simulink model "zynqRadioHWSWQPSKAD9361AD9364SL"  (R2025a)
settings: Solver=FixedStepDiscrete  StartTime=0.0  StopTime=0.5  RelTol=1e-3
PreLoadFcn:
  | setTxBurstLength = 10000;
  | txtmsg = ['Zynq radio HW/SW Co-design ÞÞÞÞ']; % Use only printable characters
  | 
  | %------------------------------------------------------------------------------------------------------
  | if ~isequal(size(txtmsg),[1 31])
  |     error('txtmsg must contain 31 characters');
  | end
  | 
  | [dataBits,msg] = zynqRadioHWSWQPSKgenHelloworldMsg(20); % generate 20 msgs for LUT
  | msgLUT = uint8(msg);
  | dataBitsLUT = dataBits(:);
  | Rsym                = 10e3;%1.92e6;
  | Config = zynqRadioHWSWQPSKTxRxParameters;
  | fs = Rsym*Config.SamplesPerSymbol;
  | word = [txtmsg newline];  % append a new line character to txtmsg
  | 
  | % The highest clock rate is 16 times the message character rate.
  | % As the message characters are fed at highest clock to FPGA
  | % repeat each character 16 times to maintain the message rate.
  | word = repelem(word.',16,1);
  | repeatTimes = ceil(setTxBurstLength/length(word));
  | inpData = complex(repmat(uint8(word),repeatTimes,1));
  | inUseTxBurstLength = length(inpData);
PostLoadFcn:
  | hScopeConfig = get_param([gcs '/HDL_QPSK/QPSK Tx Channel QPSK Rx/QPSK Rx/Frequency and Time Synchronizer/Symbol Synchronizer/No HDL/QPSK Receiver Eye Diagram'],'ScopeConfiguration');
  | hScopeConfig.OpenAtSimulationStart = false;
  | hScopeConfig.Visible = false;
  | clear hScopeConfig
InitFcn:
  | setTxBurstLength = 10000;
  | txtmsg = ['Zynq radio HW/SW Co-design ÞÞÞÞ']; % Use only printable characters
  | 
  | %------------------------------------------------------------------------------------------------------
  | if ~isequal(size(txtmsg),[1 31])
  |     error('txtmsg must contain 31 characters');
  | end
  | 
  | [dataBits,msg] = zynqRadioHWSWQPSKgenHelloworldMsg(20); % generate 20 msgs for LUT
  | msgLUT = uint8(msg);
  | dataBitsLUT = dataBits(:);
  | Rsym                = 10e3;%1.92e6;
  | Config = zynqRadioHWSWQPSKTxRxParameters;
  | fs = Rsym*Config.SamplesPerSymbol;
  | word = [txtmsg newline];  % append a new line character to txtmsg
  | 
  | % The highest clock rate is 16 times the message character rate.
  | % As the message characters are fed at highest clock to FPGA
  | % repeat each character 16 times to maintain the message rate.
  | word = repelem(word.',16,1);
  | repeatTimes = ceil(setTxBurstLength/length(word));
  | inpData = complex(repmat(uint8(word),repeatTimes,1));
  | inUseTxBurstLength = length(inpData);
  | 
  | Config.Preamble = logical(zeros(0,1))
undefined symbols (not defined in the file or in its folder): Add, dspblkCoreblockFVToolHelper, gcbh, gse_genframes, Shift
libraries: hdlsllib x144, simulink x37, dsphdlsigops2 x3, dsphdlfiltering2 x3, whdlutilities x3, dsphdlxfrm2 x2, dsphdlmathfun2 x2, commdigbbndpm3 x2, sdrzblksprivate x1
(part 4 of 6)

== system zynqRadioHWSWQPSKAD9361AD9364SL/HDL_QPSK/QPSK Tx Channel QPSK Rx/QPSK Rx/Frequency and Time Synchronizer/Preamble Detector/Timing Adjust ==
  timingOffset : Inport
  timingOffsetValid : Inport  Port=2
  dataIn : Inport  Port=3
  validIn : Inport  Port=4
  Delay{,1..4} (5 alike) : Delay  DelayLength=1
  Logical Operator : Logic  AllPortsSameDT=off  OutDataTypeStr=boolean
  Logical Operator1 : Logic  Operator=NOT  AllPortsSameDT=off  OutDataTypeStr=boolean
  Logical Operator2 : Logic  Inputs=3  AllPortsSameDT=off  OutDataTypeStr=boolean
  No HDL : Subsystem
  Relational Operator : RelationalOperator  Operator===  OutDataTypeStr=boolean  InputSameDT=off
  State Register : hdlsllib/Discrete/Unit Delay Enabled Resettable Synchronous  InitialCondition=0.0  SampleTime=-1
  Unit Delay Enabled Synchronous3 : hdlsllib/Discrete/Unit Delay Enabled Synchronous  InitialCondition=0.0  SampleTime=-1
  timing Reference : hdlsllib/Sources/HDL Counter  CountType=Count limited  CountInit=0  CountStep=1  CountMax=searchSamples - 1  CountFromType=Initial value  CountFrom=0  CountResetPort=off  CountLoadPort=off  CountEnbPort=on  CountDirPort=off  CountHitOutputPort=off  CountDataType=Unsigned  CountWordLen=nextpow2(searchSamples - 1)  CountFracLen=0  CountSampTime=1
  dataOut : Outport
  validOut : Outport  Port=2
  SyncPulse : Outport  Port=3
  wires:
  Delay4/1 -> dataOut/1
  Delay3/1 -> validOut/1
  timingOffset/1 -> Unit Delay Enabled Synchronous3/1
  Unit Delay Enabled Synchronous3/1 -> Relational Operator/2
  Delay/1 -> SyncPulse/1
  validIn/1 -> timing Reference/1, Logical Operator2/1, No HDL/1(validIn), Delay3/1
  State Register/1 -> Logical Operator2/3, Delay1/1
  Logical Operator1/1 -> Logical Operator/2
  Relational Operator/1 -> Logical Operator2/2
  Logical Operator2/1 -> No HDL/3(syncPulse), Delay/1, Delay2/1
  Delay2/1 -> State Register/3
  Logical Operator/1 -> State Register/1, State Register/2, Unit Delay Enabled Synchronous3/2
  timing Reference/1 -> No HDL/2(timingOffset), Relational Operator/1
  timingOffsetValid/1 -> Logical Operator/1
  Delay1/1 -> Logical Operator1/1
  dataIn/1 -> Delay4/1

== system zynqRadioHWSWQPSKAD9361AD9364SL/HDL_QPSK/QPSK Tx Channel QPSK Rx/QPSK Rx/Frequency and Time Synchronizer/Symbol Synchronizer/Gardner TED ==
  data : Inport
  strobe : Inport  Port=2
  Constant : Constant  Value=0  OutDataTypeStr=Inherit: Inherit via back propagation  SampleTime=1/(Rsym*SamplesPerSymbol)
  Delay10 : Delay  DelayLength=4
  GTED : Subsystem
  Switch : Switch  Criteria=u2 ~= 0  InputSameDT=off
  e : Outport  VectorParamsAs1DForOutWhenUnconnected=off
  wires:
  Constant/1 -> Switch/3
  Switch/1 -> e/1
  strobe/1 -> Delay10/1
  data/1 -> GTED/1(In1)
  GTED/1(Out1) -> Switch/1
  Delay10/1 -> Switch/2

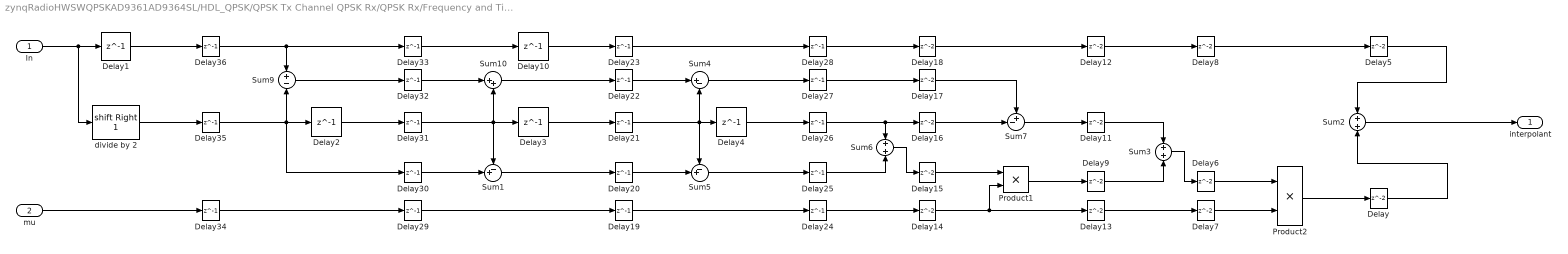
== system zynqRadioHWSWQPSKAD9361AD9364SL/HDL_QPSK/QPSK Tx Channel QPSK Rx/QPSK Rx/Frequency and Time Synchronizer/Symbol Synchronizer/Interpolation Filter ==
  In : Inport
  mu : Inport  Port=2
  Delay{,5..9,11..18} (14 alike) : Delay
  Delay{1..4,10} (5 alike) : Delay  DelayLength=1  InitialCondition=0
  Delay{19..36} (18 alike) : Delay  DelayLength=1
  Product1 : Product  OutDataTypeStr=fixdt(1,16,10)  RndMeth=Zero
  Product2 : Product  RndMeth=Zero  OutDataTypeStr=Inherit: Same as first input
  Sum1 : Sum  Inputs=-+|
  Sum10 : Sum  Inputs=|++
  Sum2 : Sum  Inputs=+|+
  Sum3 : Sum  Inputs=+|+  OutDataTypeStr=fixdt(1,16,10)
  Sum4 : Sum  Inputs=|+-
  Sum5 : Sum  Inputs=-+|
  Sum6 : Sum  Inputs=+|+  OutDataTypeStr=fixdt(1,16,11)  SaturateOnIntegerOverflow=on
  Sum7 : Sum  Inputs=+-|  OutDataTypeStr=fixdt(1,16,10)
  Sum9 : Sum  Inputs=+-
  divide by 2 : ArithShift  BitShiftNumber=1  BitShiftDirection=Right
  interpolant : Outport
  wires:
  Sum9/1 -> Delay32/1
  In/1 -> divide by 2/1, Delay1/1
  Sum2/1 -> interpolant/1
  Sum7/1 -> Delay11/1
  Product1/1 -> Delay9/1
  Product2/1 -> Delay/1
  Sum3/1 -> Delay6/1
  Sum1/1 -> Delay20/1
  Delay3/1 -> Delay21/1
  Sum10/1 -> Delay22/1
  Delay2/1 -> Delay31/1
  Delay1/1 -> Delay36/1
  divide by 2/1 -> Delay35/1
  Delay/1 -> Sum2/2
  Delay5/1 -> Sum2/1
  Delay6/1 -> Product2/1
  Delay7/1 -> Product2/2
  Delay8/1 -> Delay5/1
  Delay9/1 -> Sum3/2
  Delay11/1 -> Sum3/1
  Delay12/1 -> Delay8/1
  Delay13/1 -> Delay7/1
  Delay14/1 -> Delay13/1, Product1/2
  Delay15/1 -> Product1/1
  Delay16/1 -> Sum7/2
  Delay17/1 -> Sum7/1
  Delay18/1 -> Delay12/1
  mu/1 -> Delay34/1
  Sum5/1 -> Delay25/1
  Delay4/1 -> Delay26/1
  Sum4/1 -> Delay27/1
  Delay10/1 -> Delay23/1
  Delay24/1 -> Delay14/1
  Sum6/1 -> Delay15/1
  Delay26/1 -> Delay16/1, Sum6/1
  Delay27/1 -> Delay17/1
  Delay28/1 -> Delay18/1
  Delay25/1 -> Sum6/2
  Delay19/1 -> Delay24/1
  Delay20/1 -> Sum5/2
  Delay21/1 -> Sum4/2, Sum5/1, Delay4/1
  Delay22/1 -> Sum4/1
  Delay23/1 -> Delay28/1
  Delay29/1 -> Delay19/1
  Delay30/1 -> Sum1/2
  Delay31/1 -> Sum1/1, Sum10/2, Delay3/1
  Delay32/1 -> Sum10/1
  Delay33/1 -> Delay10/1
  Delay34/1 -> Delay29/1
  Delay35/1 -> Delay30/1, Delay2/1, Sum9/2
  Delay36/1 -> Delay33/1, Sum9/1

== system zynqRadioHWSWQPSKAD9361AD9364SL/HDL_QPSK/QPSK Tx Channel QPSK Rx/QPSK Rx/Frequency and Time Synchronizer/Symbol Synchronizer/Loop Filter ==
  note: Proportional-Plus-Integrator Loop Filter,
      | Infinite DC Response to guarantee convergence
  e : Inport
  Add : Sum
  Add2 : Sum  Inputs=|++  OutDataTypeStr=Inherit: Same as first input
  Data Type Conversion17 : DataTypeConversion  OutDataTypeStr=fixdt(1,11,10)  SaturateOnIntegerOverflow=off  RndMeth=Floor
  Delay : Delay  DelayLength=1
  Delay1 : Delay  DelayLength=1  InitialCondition=0
  Delay2 : Delay  InitialCondition=0
  Delay3 : Delay  InitialCondition=0
  Delay4 : Delay  DelayLength=1  InitialCondition=0
  Delay5 : Delay  InitialCondition=0
  Delay6 : Delay  DelayLength=1
  K1 : Gain  Gain=fi(SSLoopFilterPropGain,1,24,24)  ParamDataTypeStr=Inherit: Inherit from 'Gain'  OutDataTypeStr=fixdt(1,30,23)
  K2 : Gain  Gain=fi(SSLoopFilterIntegGain,1,24,24)  ParamDataTypeStr=Inherit: Inherit from 'Gain'  OutDataTypeStr=fixdt(1,30,23)
  v : Outport
  wires:
  Delay/1 -> Add2/2
  Delay5/1 -> Delay6/1
  Delay3/1 -> Delay1/1
  e/1 -> Delay2/1
  Add/1 -> Data Type Conversion17/1
  Delay1/1 -> Add/1
  Delay4/1 -> Add/2
  Delay2/1 -> K1/1, K2/1
  Data Type Conversion17/1 -> v/1
  K2/1 -> Delay5/1
  Add2/1 -> Delay/1, Delay4/1
  K1/1 -> Delay3/1
  Delay6/1 -> Add2/1

== system zynqRadioHWSWQPSKAD9361AD9364SL/HDL_QPSK/QPSK Tx Channel QPSK Rx/QPSK Rx/Frequency and Time Synchronizer/Symbol Synchronizer/No HDL ==
  data : Inport
  valid : Inport  Port=2
  Data Type Conversion : DataTypeConversion  OutDataTypeStr=double  SaturateOnIntegerOverflow=off  RndMeth=Floor
  No HDL : Subsystem
  QPSK Receiver Eye Diagram : EyeDiagramBlock  WindowPosition=[177.000000,528.000000,1920.000000,977.000000,]  ScopeFrameLocation=window  SamplesPerSymbol=SamplesPerSymbol  SymbolsPerTrace=1  Title=RRC Matched Filtered Output  YLimits=[-1.1602,1.2629]
      settings: OpenAtSimulationStart=off
  Unit Delay Enabled Synchronous : hdlsllib/Discrete/Unit Delay Enabled Synchronous  InitialCondition=0.0  SampleTime=-1
  wires:
  data/1 -> No HDL/1(data), Unit Delay Enabled Synchronous/1
  Data Type Conversion/1 -> QPSK Receiver Eye Diagram/1
  Unit Delay Enabled Synchronous/1 -> Data Type Conversion/1
  valid/1 -> Unit Delay Enabled Synchronous/2, No HDL/Enable

== system zynqRadioHWSWQPSKAD9361AD9364SL/HDL_QPSK/QPSK Tx Channel QPSK Rx/QPSK Rx/Frequency and Time Synchronizer/Symbol Synchronizer/Rate Handle ==
  dataIn : Inport
  strobe : Inport  Port=2
  validIn : Inport  Port=3
  Compare To Constant : simulink/Logic and Bit Operations/Compare To Constant  relop===  const=0  OutDataTypeStr=boolean
  Constant : Constant  Value=false  SampleTime=-1
  FIFO : Subsystem  mask{fifoSize=32*4, pushFullDiag=Error, popEmptyDiag=Ignore}
      mask prompts: fifoSize "FIFO size:"; pushFullDiag "Push full FIFO:"; popEmptyDiag "Pop empty FIFO:"
      mask TypeOptions pushFullDiag: Ignore | Warning | Error
      mask TypeOptions popEmptyDiag: Ignore | Warning | Error
  HDL Counter : hdlsllib/Sources/HDL Counter  CountType=Count limited  CountInit=0  CountStep=1  CountMax=SamplesPerSymbol - 1  CountFromType=Initial value  CountFrom=0  CountResetPort=off  CountLoadPort=off  CountEnbPort=on  CountDirPort=off  CountHitOutputPort=off  CountDataType=Unsigned  CountWordLen=nextpow2(SamplesPerSymbol - 1)  CountFracLen=0  CountSampTime=1
  Logical Operator : Logic  AllPortsSameDT=off  OutDataTypeStr=boolean
  Logical Operator1 : Logic  AllPortsSameDT=off  OutDataTypeStr=boolean
  Terminator : Terminator
  dataOut : Outport
  validOut : Outport  Port=2
  wires:
  dataIn/1 -> FIFO/1(in)
  validIn/1 -> Logical Operator1/2, Logical Operator/1, HDL Counter/1
  HDL Counter/1 -> Compare To Constant/1
  Compare To Constant/1 -> Logical Operator/2
  Logical Operator/1 -> FIFO/3(pop)
  FIFO/1(out) -> dataOut/1
  FIFO/3(validPop) -> validOut/1
  FIFO/2(numEntries) -> Terminator/1  "rx_fts_ss_rh_fifo_numEntries"
  Constant/1 -> FIFO/4(reset)
  strobe/1 -> Logical Operator1/1
  Logical Operator1/1 -> FIFO/2(push)

== system zynqRadioHWSWQPSKAD9361AD9364SL/HDL_QPSK/QPSK Tx Channel QPSK Rx/QPSK Tx/Bit Packetizer/Data Bits FIFO/No HDL ==
  push : Inport
  pop : Inport  Port=2
  MATLAB Function : MATLAB Function  TreatAsAtomicUnit=on
  No HDL : Subsystem
  wires:
  push/1 -> MATLAB Function/1(wr), No HDL/1(push)
  pop/1 -> MATLAB Function/2(rd), No HDL/5(pop)
  MATLAB Function/2(ncount) -> No HDL/3(ncount)
  MATLAB Function/1(full) -> No HDL/2(full)
  MATLAB Function/3(empty) -> No HDL/4(empty)

== system zynqRadioHWSWQPSKAD9361AD9364SL/HDL_QPSK/QPSK Tx Channel QPSK Rx/QPSK Tx/Bit Packetizer/Preamble Bits Generator/Preamble Bits Store ==
  note: The Preamble is padded with zeros in the LUT such that
      | the length is the 2^nextpow2(length(Preamble)) for
      | efficient resource mapping to RAM
  actualPreamble : Inport
  sampleCount : Inport  Port=2
  Constant : Constant  OutDataTypeStr=boolean  SampleTime=1/(Rsym*4)
  Extract Bits : simulink/Logic and Bit Operations/Extract Bits  bitsToExtract=Range of bits  numBits=8  bitIdxRange=[0 nextpow2(length(Preamble))-1]  outScalingMode=Treat bit field as an integer
  Preamble : LookupNDDirect  NumberOfTableDimensions=1  Table=[Preamble;false(32-length(Preamble),1)]  DiagnosticForOutOfRangeInput=Error
  Switch : Switch  Criteria=u2 ~= 0  Threshold=1  SaturateOnIntegerOverflow=off  InputSameDT=off
  preamble : Outport
  wires:
  Switch/1 -> preamble/1
  Constant/1 -> Switch/3
  Extract Bits/1 -> Preamble/1
  Preamble/1 -> Switch/1
  sampleCount/1 -> Extract Bits/1
  actualPreamble/1 -> Switch/2

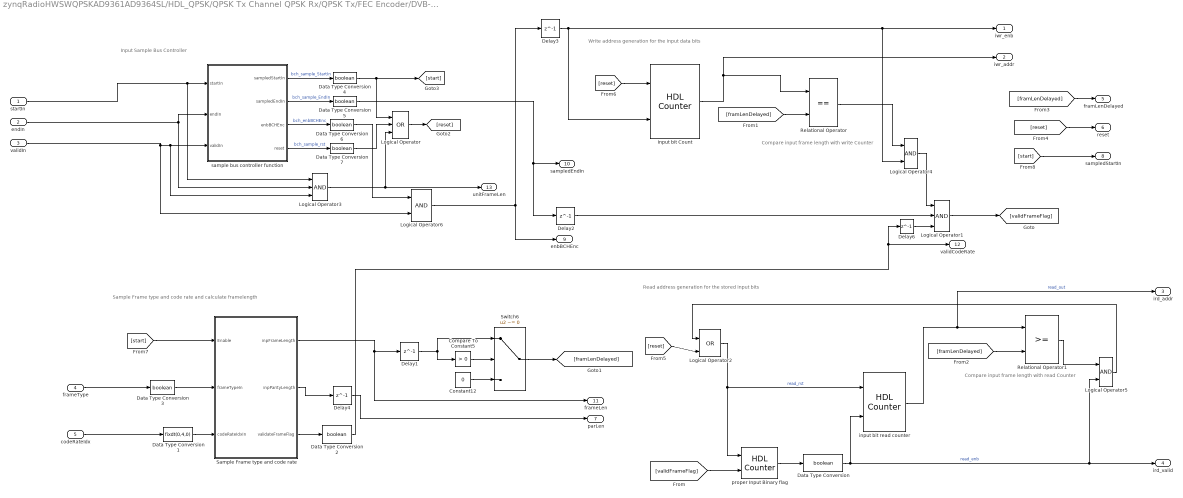
== system zynqRadioHWSWQPSKAD9361AD9364SL/HDL_QPSK/QPSK Tx Channel QPSK Rx/QPSK Tx/FEC Encoder/DVB-S2 BCH Encoder/Input controller ==
  note: Input Sample Bus Controller
  note: Compare input frame length with read Counter
  note: Compare input frame length with write Counter
  note: Sample Frame type and code rate and calculate framelength
  note: Write address generation for the input data bits
  note: Read address generation for the stored input bits
  startIn : Inport
  endIn : Inport  Port=2
  validIn : Inport  Port=3
  frameType : Inport  Port=4
  codeRateIdx : Inport  Port=5
  Compare To Constant5 : simulink/Logic and Bit Operations/Compare To Constant  relop=>  const=0  OutDataTypeStr=boolean
  Constant12 : Constant  Value=0  OutDataTypeStr=Inherit: Inherit via back propagation  SampleTime=-1
  Data Type Conversion{,2,4..7} (6 alike) : DataTypeConversion  OutDataTypeStr=boolean  SaturateOnIntegerOverflow=off  RndMeth=Floor
  Data Type Conversion1 : DataTypeConversion  OutDataTypeStr=fixdt(0,4,0)  RndMeth=Nearest  SaturateOnIntegerOverflow=off
  Data Type Conversion3 : DataTypeConversion  OutDataTypeStr=boolean  RndMeth=Nearest  SaturateOnIntegerOverflow=off
  Delay{1..4,6} (5 alike) : Delay  DelayLength=1
  Input bit Count : hdlsllib/Sources/HDL Counter  CountType=Count limited  CountInit=0  CountStep=1  CountMax=65535  CountFromType=Initial value  CountFrom=0  CountResetPort=on  CountLoadPort=off  CountEnbPort=on  CountDirPort=off  CountHitOutputPort=off  CountDataType=Unsigned  CountWordLen=16  CountFracLen=0  CountSampTime=1
  Logical Operator : Logic  Operator=OR  Inputs=3  IconShape=distinctive  AllPortsSameDT=off  OutDataTypeStr=boolean
  Logical Operator1 : Logic  Inputs=3  IconShape=distinctive  AllPortsSameDT=off  OutDataTypeStr=boolean
  Logical Operator2 : Logic  Operator=OR  IconShape=distinctive  AllPortsSameDT=off  OutDataTypeStr=boolean
  Logical Operator3 : Logic  Inputs=3  IconShape=distinctive  AllPortsSameDT=off  OutDataTypeStr=boolean
  Logical Operator4 : Logic  IconShape=distinctive  AllPortsSameDT=off  OutDataTypeStr=boolean
  Logical Operator5 : Logic  IconShape=distinctive  AllPortsSameDT=off  OutDataTypeStr=boolean
  Logical Operator6 : Logic  IconShape=distinctive  AllPortsSameDT=off  OutDataTypeStr=boolean
  Relational Operator : RelationalOperator  Operator===  OutDataTypeStr=boolean  InputSameDT=off
  Relational Operator1 : RelationalOperator  OutDataTypeStr=boolean  InputSameDT=off
  Sample Frame type and code rate : MATLAB Function  TreatAsAtomicUnit=on
  Switch6 : Switch  Criteria=u2 ~= 0  SaturateOnIntegerOverflow=off  InputSameDT=off
  input bit read counter : hdlsllib/Sources/HDL Counter  CountType=Count limited  CountInit=0  CountStep=1  CountMax=65535  CountFromType=Initial value  CountFrom=0  CountResetPort=on  CountLoadPort=off  CountEnbPort=on  CountDirPort=off  CountHitOutputPort=off  CountDataType=Unsigned  CountWordLen=16  CountFracLen=0  CountSampTime=1
  proper Input Binary flag : hdlsllib/Sources/HDL Counter  CountType=Count limited  CountInit=0  CountStep=1  CountMax=1  CountFromType=Initial value  CountFrom=0  CountResetPort=on  CountLoadPort=off  CountEnbPort=on  CountDirPort=off  CountHitOutputPort=off  CountDataType=Unsigned  CountWordLen=1  CountFracLen=0  CountSampTime=1
  sample bus controller function : MATLAB Function  TreatAsAtomicUnit=on
  iwr_enb : Outport
  iwr_addr : Outport  Port=2
  ird_addr : Outport  Port=3
  ird_valid : Outport  Port=4
  framLenDelayed : Outport  Port=5
  reset : Outport  Port=6
  parLen : Outport  Port=7
  sampledStartIn : Outport  Port=8
  enbBCHEnc : Outport  Port=9
  sampledEndIn : Outport  Port=10
  frameLen : Outport  Port=11
  validCodeRate : Outport  Port=12
  unitFrameLen : Outport  Port=13
  wires:
  Input bit Count/1 -> iwr_addr/1, Relational Operator/1
  Data Type Conversion2/1 -> Delay6/1, validCodeRate/1
  input bit read counter/1 -> ird_addr/1, Relational Operator1/1  "read_out"
  Data Type Conversion/1 -> input bit read counter/2, Logical Operator5/2, ird_valid/1  "read_enb"
  Sample Frame type and code rate/1(inpFrameLength) -> frameLen/1, Delay1/1
  Delay3/1 -> iwr_enb/1, Logical Operator4/2, Input bit Count/2
  Logical Operator3/1 -> Logical Operator/3, unitFrameLen/1
  Delay4/1 -> parLen/1
  [validFrameFlag] -> proper Input Binary flag/2
  Delay6/1 -> Logical Operator1/3
  Sample Frame type and code rate/3(validateFrameFlag) -> Data Type Conversion2/1
  Relational Operator1/1 -> Logical Operator5/1
  Relational Operator/1 -> Logical Operator4/1
  Sample Frame type and code rate/2(inpParityLength) -> Delay4/1
  Logical Operator5/1 -> Logical Operator2/1
  Logical Operator2/1 -> proper Input Binary flag/1, input bit read counter/1  "read_rst"
  proper Input Binary flag/1 -> Data Type Conversion/1
  Logical Operator1/1 -> [validFrameFlag]
  Delay2/1 -> Logical Operator1/2
  Data Type Conversion5/1 -> Delay2/1, sampledEndIn/1
  Delay1/1 -> Compare To Constant5/1, Switch6/1
  Data Type Conversion4/1 -> [start], Logical Operator/1
  Logical Operator6/1 -> enbBCHEnc/1, Delay3/1
  codeRateIdx/1 -> Data Type Conversion1/1
  frameType/1 -> Data Type Conversion3/1
  Data Type Conversion1/1 -> Sample Frame type and code rate/3(codeRateIdxIn)
  Logical Operator4/1 -> Logical Operator1/1
  Data Type Conversion3/1 -> Sample Frame type and code rate/2(frameTypeIn)
  Constant12/1 -> Switch6/3
  Compare To Constant5/1 -> Switch6/2
  Data Type Conversion6/1 -> Logical Operator6/1
  Data Type Conversion7/1 -> Logical Operator/2
  startIn/1 -> Logical Operator3/1, sample bus controller function/1(startIn)
  validIn/1 -> Logical Operator6/2, Logical Operator3/3, sample bus controller function/3(validIn)
  sample bus controller function/2(sampledEndIn) -> Data Type Conversion5/1  "bch_sample_EndIn"
  sample bus controller function/3(enbBCHEnc) -> Data Type Conversion6/1  "bch_enbBCHEnc"
  endIn/1 -> sample bus controller function/2(endIn), Logical Operator3/2
  sample bus controller function/4(reset) -> Data Type Conversion7/1  "bch_sample_rst"
  sample bus controller function/1(sampledStartIn) -> Data Type Conversion4/1  "bch_sample_StartIn"
  Switch6/1 -> [framLenDelayed]
  [framLenDelayed] -> Relational Operator/2
  [framLenDelayed] -> Relational Operator1/2
  [framLenDelayed] -> framLenDelayed/1
  Logical Operator/1 -> [reset]
  [reset] -> reset/1
  [reset] -> Logical Operator2/2
  [reset] -> Input bit Count/1
  [start] -> Sample Frame type and code rate/1(Enable)
  [start] -> sampledStartIn/1

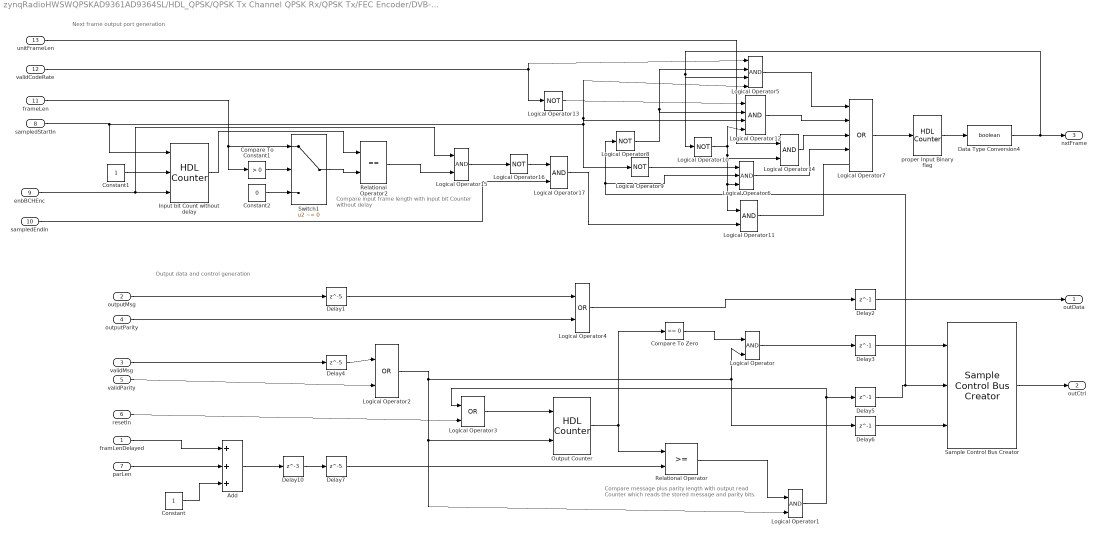
== system zynqRadioHWSWQPSKAD9361AD9364SL/HDL_QPSK/QPSK Tx Channel QPSK Rx/QPSK Tx/FEC Encoder/DVB-S2 BCH Encoder/Output Controller ==
  note: Output data and control generation
  note: Next frame output port generation
  note: Compare message plus parity length with output read Counter which reads the stored message and parity bits.
  note: Compare input frame length with input bit Counter without delay
  framLenDelayed : Inport
  outputMsg : Inport  Port=2
  validMsg : Inport  Port=3
  outputParity : Inport  Port=4
  validParity : Inport  Port=5
  resetIn : Inport  Port=6
  parLen : Inport  Port=7
  sampledStartIn : Inport  Port=8
  enbBCHEnc : Inport  Port=9
  sampledEndIn : Inport  Port=10
  frameLen : Inport  Port=11
  validCodeRate : Inport  Port=12
  unitFrameLen : Inport  Port=13
  Add : Sum  Inputs=+++  OutDataTypeStr=Inherit: Same as first input
  Compare To Constant1 : simulink/Logic and Bit Operations/Compare To Constant  relop=>  const=0  OutDataTypeStr=boolean
  Compare To Zero : hdlsllib/Logic and Bit Operations/Compare To Zero  relop===  OutDataTypeStr=boolean
  Constant : Constant  OutDataTypeStr=Inherit: Inherit via back propagation  SampleTime=-1
  Constant1 : Constant  OutDataTypeStr=uint16  SampleTime=-1
  Constant2 : Constant  Value=0  OutDataTypeStr=Inherit: Inherit via back propagation  SampleTime=-1
  Data Type Conversion4 : DataTypeConversion  OutDataTypeStr=boolean  SaturateOnIntegerOverflow=off  RndMeth=Floor
  Delay1 : Delay  DelayLength=5
  Delay10 : Delay  DelayLength=3
  Delay{2..3,5..6} (4 alike) : Delay  DelayLength=1
  Delay4 : Delay  DelayLength=5
  Delay7 : Delay  DelayLength=5
  "Input bit Count without delay " : hdlsllib/Sources/HDL Counter  CountType=Count limited  CountInit=0  CountStep=1  CountMax=65535  CountFromType=Initial value  CountFrom=0  CountResetPort=off  CountLoadPort=on  CountEnbPort=on  CountDirPort=off  CountHitOutputPort=off  CountDataType=Unsigned  CountWordLen=16  CountFracLen=0  CountSampTime=1
  Logical Operator{,1,11,14..15,17} (6 alike) : Logic  IconShape=distinctive  AllPortsSameDT=off  OutDataTypeStr=boolean
  Logical Operator{8..10,13,16} (5 alike) : Logic  Operator=NOT  IconShape=distinctive  AllPortsSameDT=off  OutDataTypeStr=boolean
  Logical Operator12 : Logic  Inputs=4  IconShape=distinctive  AllPortsSameDT=off  OutDataTypeStr=boolean
  Logical Operator2 : Logic  Operator=OR  IconShape=distinctive  AllPortsSameDT=off  OutDataTypeStr=boolean
  Logical Operator3 : Logic  Operator=OR  IconShape=distinctive  AllPortsSameDT=off  OutDataTypeStr=boolean
  Logical Operator4 : Logic  Operator=OR  IconShape=distinctive  AllPortsSameDT=off  OutDataTypeStr=boolean
  Logical Operator5 : Logic  Inputs=4  IconShape=distinctive  AllPortsSameDT=off  OutDataTypeStr=boolean
  Logical Operator6 : Logic  Inputs=3  IconShape=distinctive  AllPortsSameDT=off  OutDataTypeStr=boolean
  Logical Operator7 : Logic  Operator=OR  Inputs=5  IconShape=distinctive  AllPortsSameDT=off  OutDataTypeStr=boolean
  Output Counter : hdlsllib/Sources/HDL Counter  CountType=Count limited  CountInit=0  CountStep=1  CountMax=65535  CountFromType=Initial value  CountFrom=0  CountResetPort=on  CountLoadPort=off  CountEnbPort=on  CountDirPort=off  CountHitOutputPort=off  CountDataType=Unsigned  CountWordLen=16  CountFracLen=0  CountSampTime=1
  Relational Operator : RelationalOperator  OutDataTypeStr=boolean  InputSameDT=off
  Relational Operator2 : RelationalOperator  Operator===  OutDataTypeStr=boolean  InputSameDT=off
  Sample Control Bus Creator : whdlutilities/Sample Control Bus Creator
  Switch1 : Switch  Criteria=u2 ~= 0  SaturateOnIntegerOverflow=off  InputSameDT=off
  proper Input Binary flag : hdlsllib/Sources/HDL Counter  CountType=Count limited  CountInit=1  CountStep=1  CountMax=0  CountFromType=Initial value  CountFrom=1  CountResetPort=off  CountLoadPort=off  CountEnbPort=on  CountDirPort=off  CountHitOutputPort=off  CountDataType=Unsigned  CountWordLen=1  CountFracLen=0  CountSampTime=1
  outData : Outport
  outCtrl : Outport  Port=2
  nxtFrame : Outport  Port=3
  wires:
  Logical Operator/1 -> Delay3/1
  Logical Operator4/1 -> Delay2/1
  Sample Control Bus Creator/1 -> outCtrl/1
  resetIn/1 -> Logical Operator3/2
  Output Counter/1 -> Relational Operator/1, Compare To Zero/1
  Compare To Zero/1 -> Logical Operator/1
  Logical Operator3/1 -> Output Counter/1
  Logical Operator1/1 -> Logical Operator3/1, Delay5/1
  Relational Operator/1 -> Logical Operator1/1
  validParity/1 -> Logical Operator2/2
  Logical Operator2/1 -> Logical Operator1/2, Output Counter/2, Delay6/1, Logical Operator/2
  outputParity/1 -> Logical Operator4/2
  Delay1/1 -> Logical Operator4/1
  Delay4/1 -> Logical Operator2/1
  Delay2/1 -> outData/1
  Delay3/1 -> Sample Control Bus Creator/1
  Delay5/1 -> Logical Operator6/2, Logical Operator8/1, Sample Control Bus Creator/2
  Delay6/1 -> Sample Control Bus Creator/3
  Delay7/1 -> Relational Operator/2
  proper Input Binary flag/1 -> Data Type Conversion4/1
  Data Type Conversion4/1 -> nxtFrame/1, Logical Operator10/1, Logical Operator5/3
  Logical Operator7/1 -> proper Input Binary flag/1
  Logical Operator8/1 -> Logical Operator12/2, Logical Operator5/2
  Logical Operator9/1 -> Logical Operator6/1
  Logical Operator10/1 -> Logical Operator12/4, Logical Operator14/2, Logical Operator11/1, Logical Operator6/3
  Logical Operator6/1 -> Logical Operator7/4
  Logical Operator5/1 -> Logical Operator7/1
  outputMsg/1 -> Delay1/1
  validMsg/1 -> Delay4/1
  Delay10/1 -> Delay7/1
  Logical Operator17/1 -> Logical Operator11/2
  Logical Operator11/1 -> Logical Operator7/5
  validCodeRate/1 -> Logical Operator5/1, Logical Operator13/1
  Logical Operator12/1 -> Logical Operator7/2
  Logical Operator13/1 -> Logical Operator12/1
  parLen/1 -> Add/2
  unitFrameLen/1 -> Logical Operator14/1
  Logical Operator14/1 -> Logical Operator7/3
  Constant/1 -> Add/3
  framLenDelayed/1 -> Add/1
  Add/1 -> Delay10/1
  sampledStartIn/1 -> "Input bit Count without delay "/1, Logical Operator5/4, Logical Operator12/3, Logical Operator9/1
  enbBCHEnc/1 -> Logical Operator15/1, "Input bit Count without delay "/3
  frameLen/1 -> Compare To Constant1/1, Switch1/1
  Constant1/1 -> "Input bit Count without delay "/2
  Relational Operator2/1 -> Logical Operator15/2
  Compare To Constant1/1 -> Switch1/2
  Constant2/1 -> Switch1/3
  Logical Operator16/1 -> Logical Operator17/1
  sampledEndIn/1 -> Logical Operator17/2
  "Input bit Count without delay "/1 -> Relational Operator2/1
  Switch1/1 -> Relational Operator2/2
  Logical Operator15/1 -> Logical Operator16/1

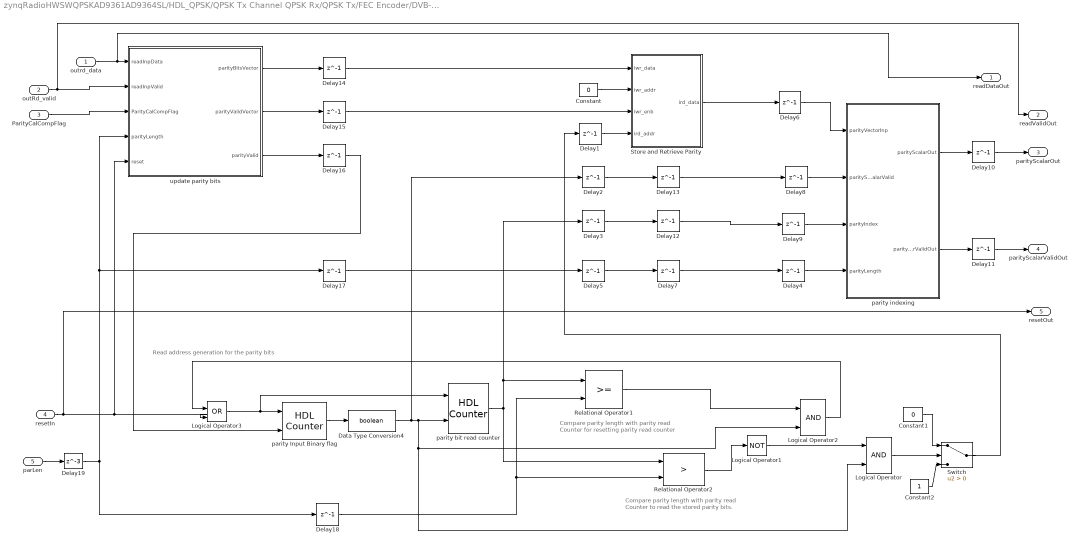
== system zynqRadioHWSWQPSKAD9361AD9364SL/HDL_QPSK/QPSK Tx Channel QPSK Rx/QPSK Tx/FEC Encoder/DVB-S2 BCH Encoder/Parity Generation ==
  note: Read address generation for the parity bits
  note: Compare parity length with parity read Counter for resetting parity read counter
  note: Compare parity length with parity read Counter to read the stored parity bits.
  outrd_data : Inport
  outRd_valid : Inport  Port=2
  ParityCalCompFlag : Inport  Port=3
  resetIn : Inport  Port=4
  parLen : Inport  Port=5
  Constant : Constant  Value=0  VectorParams1D=off  OutDataTypeStr=fixdt(0,3,0)  SampleTime=-1
  Constant1 : Constant  Value=0  VectorParams1D=off  OutDataTypeStr=fixdt(0,3,0)  SampleTime=-1
  Constant2 : Constant  VectorParams1D=off  OutDataTypeStr=fixdt(0,3,0)  SampleTime=-1
  Data Type Conversion4 : DataTypeConversion  OutDataTypeStr=boolean  SaturateOnIntegerOverflow=off  RndMeth=Floor
  Delay{1..18} (18 alike) : Delay  DelayLength=1
  Delay19 : Delay  DelayLength=3
  Logical Operator : Logic  IconShape=distinctive  AllPortsSameDT=off  OutDataTypeStr=boolean
  Logical Operator1 : Logic  Operator=NOT  IconShape=distinctive  AllPortsSameDT=off  OutDataTypeStr=boolean
  Logical Operator2 : Logic  IconShape=distinctive  AllPortsSameDT=off  OutDataTypeStr=boolean
  Logical Operator3 : Logic  Operator=OR  IconShape=distinctive  AllPortsSameDT=off  OutDataTypeStr=boolean
  Relational Operator1 : RelationalOperator  OutDataTypeStr=boolean  InputSameDT=off
  Relational Operator2 : RelationalOperator  Operator=>  OutDataTypeStr=boolean  InputSameDT=off
  Store and Retrieve Parity : Subsystem  TreatAsAtomicUnit=on
      settings: LibrarySourceBlock=|
      | hdlsllib/Ports &
      | Subsystems/For Each
      | Subsystem
  Switch : Switch  Criteria=u2 > Threshold  SaturateOnIntegerOverflow=off  InputSameDT=off
  parity Input Binary flag : hdlsllib/Sources/HDL Counter  CountType=Count limited  CountInit=0  CountStep=1  CountMax=1  CountFromType=Initial value  CountFrom=0  CountResetPort=on  CountLoadPort=off  CountEnbPort=on  CountDirPort=off  CountHitOutputPort=off  CountDataType=Unsigned  CountWordLen=1  CountFracLen=0  CountSampTime=1
  parity bit read counter : hdlsllib/Sources/HDL Counter  CountType=Count limited  CountInit=0  CountStep=1  CountMax=255  CountFromType=Initial value  CountFrom=0  CountResetPort=on  CountLoadPort=off  CountEnbPort=on  CountDirPort=off  CountHitOutputPort=off  CountDataType=Unsigned  CountWordLen=8  CountFracLen=0  CountSampTime=1
  parity indexing : MATLAB Function  TreatAsAtomicUnit=on
  update parity bits : MATLAB Function  TreatAsAtomicUnit=on
  readDataOut : Outport
  readValidOut : Outport  Port=2
  parityScalarOut : Outport  Port=3
  parityScalarValidOut : Outport  Port=4
  resetOut : Outport  Port=5
  wires:
  Logical Operator1/1 -> Logical Operator/1
  parity Input Binary flag/1 -> Data Type Conversion4/1
  Relational Operator1/1 -> Logical Operator2/1
  Logical Operator3/1 -> parity Input Binary flag/1, parity bit read counter/1
  Constant2/1 -> Switch/3
  Constant1/1 -> Switch/1
  Logical Operator2/1 -> Logical Operator3/1
  Relational Operator2/1 -> Logical Operator1/1
  Logical Operator/1 -> Switch/2
  Delay10/1 -> parityScalarOut/1
  Delay11/1 -> parityScalarValidOut/1
  update parity bits/3(parityValid) -> Delay16/1
  update parity bits/1(parityBitsVector) -> Delay14/1
  outRd_valid/1 -> readValidOut/1, update parity bits/2(readInpValid)
  outrd_data/1 -> readDataOut/1, update parity bits/1(readInpData)
  Store and Retrieve Parity/1(ird_data) -> Delay6/1
  Constant/1 -> Store and Retrieve Parity/2(iwr_addr)
  update parity bits/2(parityValidVector) -> Delay15/1
  ParityCalCompFlag/1 -> update parity bits/3(ParityCalCompFlag)
  Switch/1 -> Delay1/1
  parity indexing/2(parityScalarValidOut) -> Delay11/1
  parity indexing/1(parityScalarOut) -> Delay10/1
  parLen/1 -> Delay19/1
  parity bit read counter/1 -> Relational Operator1/1, Delay3/1, Relational Operator2/1
  Data Type Conversion4/1 -> Logical Operator/2, Logical Operator2/2, parity bit read counter/2, Delay2/1
  resetIn/1 -> resetOut/1, update parity bits/5(reset), Logical Operator3/2
  Delay1/1 -> Store and Retrieve Parity/4(ird_addr)
  Delay2/1 -> Delay13/1
  Delay3/1 -> Delay12/1
  Delay4/1 -> parity indexing/4(parityLength)
  Delay5/1 -> Delay7/1
  Delay6/1 -> parity indexing/1(parityVectorInp)
  Delay7/1 -> Delay4/1
  Delay8/1 -> parity indexing/2(parityScalarValid)
  Delay9/1 -> parity indexing/3(parityIndex)
  Delay13/1 -> Delay8/1
  Delay12/1 -> Delay9/1
  Delay14/1 -> Store and Retrieve Parity/1(iwr_data)
  Delay15/1 -> Store and Retrieve Parity/3(iwr_enb)
  Delay16/1 -> parity Input Binary flag/2
  Delay17/1 -> Delay5/1
  Delay18/1 -> Relational Operator1/2, Relational Operator2/2
  Delay19/1 -> Delay18/1, Delay17/1, update parity bits/4(parityLength)

== system zynqRadioHWSWQPSKAD9361AD9364SL/HDL_QPSK/QPSK Tx Channel QPSK Rx/QPSK Tx/FEC Encoder/DVB-S2 BCH Encoder/Store and Retreive Input ==
  note: write and read input data using RAM
  note: Compare input frame length with read Counter
  iwr_data : Inport
  iwr_enb : Inport  Port=2
  iwr_addr : Inport  Port=3
  ird_addr : Inport  Port=4
  ird_valid : Inport  Port=5
  framLenDelayed : Inport  Port=6
  resetIn : Inport  Port=7
  Constant : Constant  Value=0  OutDataTypeStr=Inherit: Inherit via back propagation  SampleTime=-1
  Constant2 : Constant  Value=0  OutDataTypeStr=Inherit: Inherit via back propagation  SampleTime=-1
  Data RAM : hdlsllib/HDL RAMs/Simple Dual Port RAM  ram_size=16
  Data Type Duplicate : DataTypeDuplicate
  Data Type Duplicate1 : DataTypeDuplicate
  Data Type Conversion : DataTypeConversion  OutDataTypeStr=boolean  SaturateOnIntegerOverflow=off  RndMeth=Floor
  Delay{,1..3,7} (5 alike) : Delay  DelayLength=1
  Delay4 : Delay
  Delay5 : Delay
  Delay6 : Delay
  Logical Operator : Logic  Operator=NOT  IconShape=distinctive  AllPortsSameDT=off  OutDataTypeStr=boolean
  Logical Operator1 : Logic  IconShape=distinctive  AllPortsSameDT=off  OutDataTypeStr=boolean
  Logical Operator2 : Logic  IconShape=distinctive  AllPortsSameDT=off  OutDataTypeStr=boolean
  Relational Operator1 : RelationalOperator  OutDataTypeStr=boolean  InputSameDT=off
  Switch : Switch  Criteria=u2 > Threshold  SaturateOnIntegerOverflow=off  InputSameDT=off
  Switch1 : Switch  Criteria=u2 ~= 0  SaturateOnIntegerOverflow=off  InputSameDT=off
  framLenDelay : Outport
  outrd_data : Outport  Port=2
  outRd_valid : Outport  Port=3
  ParityCalCompFlag : Outport  Port=4
  resetOut : Outport  Port=5
  wires:
  Data RAM/1 -> Delay4/1
  iwr_data/1 -> Delay7/1
  ird_valid/1 -> Delay/1
  framLenDelayed/1 -> framLenDelay/1, Delay2/1
  Delay1/1 -> Relational Operator1/1
  Delay2/1 -> Relational Operator1/2
  Relational Operator1/1 -> Logical Operator1/1
  Logical Operator1/1 -> Delay6/1
  resetIn/1 -> resetOut/1, Logical Operator/1
  Logical Operator/1 -> Delay3/1
  Logical Operator2/1 -> Delay5/1, Logical Operator1/2
  Delay/1 -> Logical Operator2/1
  Delay3/1 -> Logical Operator2/2
  Switch/1 -> outrd_data/1
  Delay5/1 -> Switch/2, outRd_valid/1
  Delay6/1 -> ParityCalCompFlag/1
  Delay4/1 -> Switch/1, Data Type Duplicate/1
  Constant/1 -> Switch/3, Data Type Duplicate/2
  Switch1/1 -> Data RAM/1
  ird_addr/1 -> Data RAM/4, Delay1/1
  iwr_enb/1 -> Data RAM/3, Switch1/2
  iwr_addr/1 -> Data RAM/2
  Data Type Conversion/1 -> Switch1/1, Data Type Duplicate1/1
  Constant2/1 -> Data Type Duplicate1/2, Switch1/3
  Delay7/1 -> Data Type Conversion/1

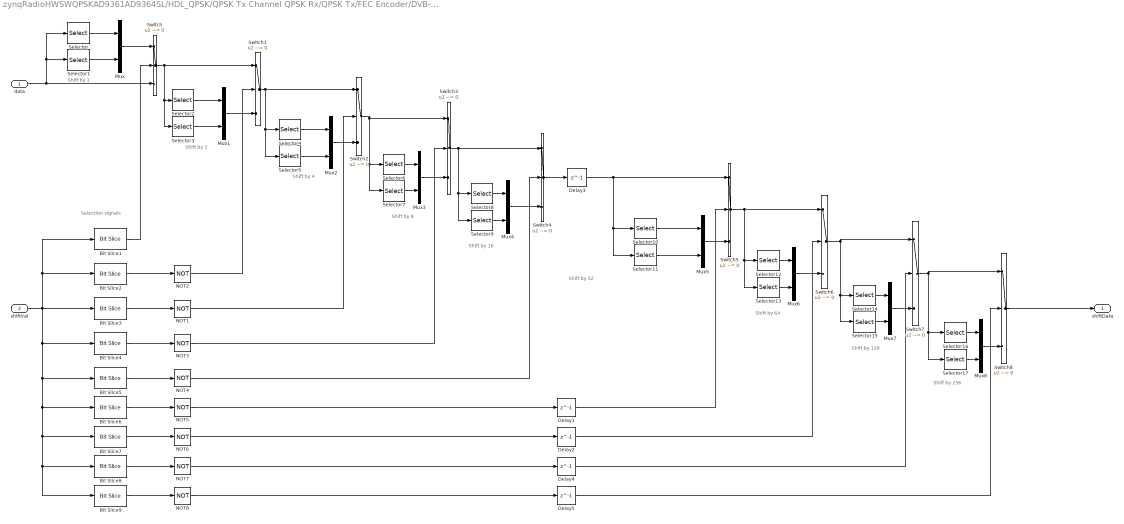
== system zynqRadioHWSWQPSKAD9361AD9364SL/HDL_QPSK/QPSK Tx Channel QPSK Rx/QPSK Tx/FEC Encoder/DVB-S2 LDPC Encoder/Circular Shifter ==
  note: Shift by 256
  note: Shift by 128
  note: Shift by 64
  note: Shift by 32
  note: Shift by 16
  note: Shift by 8
  note: Shift by 4
  note: Shift by 2
  note: Shift by 1
  note: Selection signals
  data : Inport
  shiftVal : Inport  Port=2
  Bit Slice1 : hdlsllib/Logic and Bit Operations/Bit Slice  lidx=0  ridx=0
  Bit Slice2 : hdlsllib/Logic and Bit Operations/Bit Slice  lidx=1  ridx=1
  Bit Slice3 : hdlsllib/Logic and Bit Operations/Bit Slice  lidx=2  ridx=2
  Bit Slice4 : hdlsllib/Logic and Bit Operations/Bit Slice  lidx=3  ridx=3
  Bit Slice5 : hdlsllib/Logic and Bit Operations/Bit Slice  lidx=4  ridx=4
  Bit Slice6 : hdlsllib/Logic and Bit Operations/Bit Slice  lidx=5  ridx=5
  Bit Slice7 : hdlsllib/Logic and Bit Operations/Bit Slice  lidx=6  ridx=6
  Bit Slice8 : hdlsllib/Logic and Bit Operations/Bit Slice  lidx=7  ridx=7
  Bit Slice9 : hdlsllib/Logic and Bit Operations/Bit Slice  lidx=8  ridx=8
  Delay{1..5} (5 alike) : Delay  DelayLength=1
  Mux{,1..8} (9 alike) : Mux  Inputs=2
  NOT{1..8} (8 alike) : Logic  Operator=NOT  IconShape=distinctive  AllPortsSameDT=off  OutDataTypeStr=boolean
  Selector : Selector  InputPortWidth=360  IndexOptions=Index vector (dialog)  Indices=[2 : 360]  OutputSizes=1
  Selector1 : Selector  InputPortWidth=360  IndexOptions=Index vector (dialog)  Indices=[1]  OutputSizes=1
  Selector10 : Selector  InputPortWidth=360  IndexOptions=Index vector (dialog)  Indices=[33: 360]  OutputSizes=1
  Selector11 : Selector  InputPortWidth=360  IndexOptions=Index vector (dialog)  Indices=[1:32]  OutputSizes=1
  Selector12 : Selector  InputPortWidth=360  IndexOptions=Index vector (dialog)  Indices=[65: 360]  OutputSizes=1
  Selector13 : Selector  InputPortWidth=360  IndexOptions=Index vector (dialog)  Indices=[1:64]  OutputSizes=1
  Selector14 : Selector  InputPortWidth=360  IndexOptions=Index vector (dialog)  Indices=[129: 360]  OutputSizes=1
  Selector15 : Selector  InputPortWidth=360  IndexOptions=Index vector (dialog)  Indices=[1:128]  OutputSizes=1
  Selector16 : Selector  InputPortWidth=360  IndexOptions=Index vector (dialog)  Indices=[257: 360]  OutputSizes=1
  Selector17 : Selector  InputPortWidth=360  IndexOptions=Index vector (dialog)  Indices=[1:256]  OutputSizes=1
  Selector2 : Selector  InputPortWidth=360  IndexOptions=Index vector (dialog)  Indices=[3 : 360]  OutputSizes=1
  Selector3 : Selector  InputPortWidth=360  IndexOptions=Index vector (dialog)  Indices=[1:2]  OutputSizes=1
  Selector4 : Selector  InputPortWidth=360  IndexOptions=Index vector (dialog)  Indices=[5 : 360]  OutputSizes=1
  Selector5 : Selector  InputPortWidth=360  IndexOptions=Index vector (dialog)  Indices=[1:4]  OutputSizes=1
  Selector6 : Selector  InputPortWidth=360  IndexOptions=Index vector (dialog)  Indices=[9 : 360]  OutputSizes=1
  Selector7 : Selector  InputPortWidth=360  IndexOptions=Index vector (dialog)  Indices=[1:8]  OutputSizes=1
  Selector8 : Selector  InputPortWidth=360  IndexOptions=Index vector (dialog)  Indices=[17 : 360]  OutputSizes=1
  Selector9 : Selector  InputPortWidth=360  IndexOptions=Index vector (dialog)  Indices=[1:16]  OutputSizes=1
  Switch{,1..8} (9 alike) : Switch  Criteria=u2 ~= 0  InputSameDT=off
  shiftData : Outport
  wires:
  Delay5/1 -> Switch8/2
  Delay4/1 -> Switch7/2
  Delay2/1 -> Switch6/2
  Delay1/1 -> Switch5/2
  Delay3/1 -> Switch5/1, Selector10/1, Selector11/1
  NOT8/1 -> Delay5/1
  NOT7/1 -> Delay4/1
  NOT6/1 -> Delay2/1
  NOT5/1 -> Delay1/1
  Switch4/1 -> Delay3/1
  NOT4/1 -> Switch4/2
  NOT3/1 -> Switch3/2
  NOT1/1 -> Switch2/2
  NOT2/1 -> Switch1/2
  Bit Slice1/1 -> Switch/2
  Bit Slice9/1 -> NOT8/1
  Bit Slice8/1 -> NOT7/1
  Bit Slice7/1 -> NOT6/1
  Bit Slice6/1 -> NOT5/1
  Bit Slice5/1 -> NOT4/1
  Bit Slice4/1 -> NOT3/1
  Bit Slice3/1 -> NOT1/1
  Bit Slice2/1 -> NOT2/1
  Mux8/1 -> Switch8/3
  Switch7/1 -> Switch8/1, Selector17/1, Selector16/1
  Selector16/1 -> Mux8/1
  Selector17/1 -> Mux8/2
  Mux7/1 -> Switch7/3
  Selector15/1 -> Mux7/2
  Switch6/1 -> Switch7/1, Selector15/1, Selector14/1
  Selector14/1 -> Mux7/1
  Mux6/1 -> Switch6/3
  Switch5/1 -> Switch6/1, Selector13/1, Selector12/1
  Selector13/1 -> Mux6/2
  Selector12/1 -> Mux6/1
  Selector10/1 -> Mux5/1
  Mux5/1 -> Switch5/3
  Selector11/1 -> Mux5/2
  Mux4/1 -> Switch4/3
  Selector8/1 -> Mux4/1
  Switch3/1 -> Selector9/1, Selector8/1, Switch4/1
  Selector9/1 -> Mux4/2
  Mux3/1 -> Switch3/3
  Switch2/1 -> Switch3/1, Selector7/1, Selector6/1
  Selector7/1 -> Mux3/2
  Selector6/1 -> Mux3/1
  Switch1/1 -> Selector5/1, Selector4/1, Switch2/1
  Selector4/1 -> Mux2/1
  Mux2/1 -> Switch2/3
  Selector5/1 -> Mux2/2
  Mux1/1 -> Switch1/3
  Switch/1 -> Switch1/1, Selector2/1, Selector3/1
  Selector2/1 -> Mux1/1
  Selector3/1 -> Mux1/2
  Selector1/1 -> Mux/2
  Selector/1 -> Mux/1
  Mux/1 -> Switch/1
  data/1 -> Switch/3, Selector1/1, Selector/1
  shiftVal/1 -> Bit Slice9/1, Bit Slice8/1, Bit Slice7/1, Bit Slice6/1, Bit Slice5/1, Bit Slice4/1, Bit Slice3/1, Bit Slice2/1, Bit Slice1/1
  Switch8/1 -> shiftData/1

== system zynqRadioHWSWQPSKAD9361AD9364SL/HDL_QPSK/QPSK Tx Channel QPSK Rx/QPSK Tx/FEC Encoder/DVB-S2 LDPC Encoder/Input RAM ==
  iwr_data : Inport
  iwr_addr : Inport  Port=2
  iwr_enb : Inport  Port=3
  ird_addr : Inport  Port=4
  AND : Logic  IconShape=distinctive  AllPortsSameDT=off  OutDataTypeStr=boolean
  ConvertToMux : MATLAB Function  TreatAsAtomicUnit=on
  ConvertToWord : MATLAB Function  TreatAsAtomicUnit=on
  Data Type Conversion{,1..3} (4 alike) : DataTypeConversion  OutDataTypeStr=fixdt(0,1,0)  SaturateOnIntegerOverflow=off  RndMeth=Floor
  Delay : Delay  DelayLength=1
  Delay1 : Delay  DelayLength=1
  Dual Port RAM System{,1..3} (4 alike) : hdlsllib/HDL RAMs/Dual Port RAM System  RAMType=Simple dual port  AsyncRead=off  WriteOutputValue=New data  RAMInitialValue=0  allowBusInputs=off  WritesHaveOutput=on  NumReads=0  NumWrites=1  SimulateUsing=Code generation  ModelRAMDelay=on  VectorAccess=Parallel
  Mux : Mux
  Relational Operator : RelationalOperator  Operator===  OutDataTypeStr=boolean  RndMeth=Simplest  InputSameDT=off
  Selector : Selector  InputPortWidth=360  IndexOptions=Index vector (dialog)  Indices=[1:90]  OutputSizes=1
  Selector1 : Selector  InputPortWidth=360  IndexOptions=Index vector (dialog)  Indices=[91:180]  OutputSizes=1
  Selector2 : Selector  InputPortWidth=360  IndexOptions=Index vector (dialog)  Indices=[181:270]  OutputSizes=1
  Selector3 : Selector  InputPortWidth=360  IndexOptions=Index vector (dialog)  Indices=[271:360]  OutputSizes=1
  Switch : Switch  Criteria=u2 > Threshold  SaturateOnIntegerOverflow=off  InputSameDT=off
  ird_data : Outport
  wires:
  Mux/1 -> Switch/3
  ConvertToMux/3(y3) -> Mux/3
  Dual Port RAM System1/1 -> ConvertToMux/2(u2)
  ConvertToMux/1(y1) -> Mux/1
  ConvertToWord/2(y2) -> Dual Port RAM System1/1
  ConvertToWord/4(y4) -> Dual Port RAM System2/1
  ird_addr/1 -> Dual Port RAM System/4, Relational Operator/2, Dual Port RAM System1/4, Dual Port RAM System3/4, Dual Port RAM System2/4
  Data Type Conversion2/1 -> ConvertToWord/3(u3)
  Dual Port RAM System3/1 -> ConvertToMux/3(u3)
  Delay1/1 -> AND/2
  Data Type Conversion/1 -> ConvertToWord/1(u1)
  Selector/1 -> Data Type Conversion/1
  Switch/1 -> ird_data/1
  Data Type Conversion1/1 -> ConvertToWord/2(u2)
  Delay/1 -> Switch/1
  ConvertToWord/1(y1) -> Dual Port RAM System/1
  AND/1 -> Switch/2
  ConvertToMux/4(y4) -> Mux/4
  iwr_addr/1 -> Dual Port RAM System/2, Dual Port RAM System1/2, Dual Port RAM System2/2, Dual Port RAM System3/2, Relational Operator/1
  Data Type Conversion3/1 -> ConvertToWord/4(u4)
  Dual Port RAM System2/1 -> ConvertToMux/4(u4)
  iwr_enb/1 -> Dual Port RAM System/3, Dual Port RAM System1/3, Dual Port RAM System3/3, Dual Port RAM System2/3, Delay1/1
  Selector2/1 -> Data Type Conversion2/1
  ConvertToWord/3(y3) -> Dual Port RAM System3/1
  Dual Port RAM System/1 -> ConvertToMux/1(u1)
  ConvertToMux/2(y2) -> Mux/2
  Relational Operator/1 -> AND/1
  iwr_data/1 -> Selector/1, Selector1/1, Selector2/1, Selector3/1, Delay/1
  Selector3/1 -> Data Type Conversion3/1
  Selector1/1 -> Data Type Conversion1/1

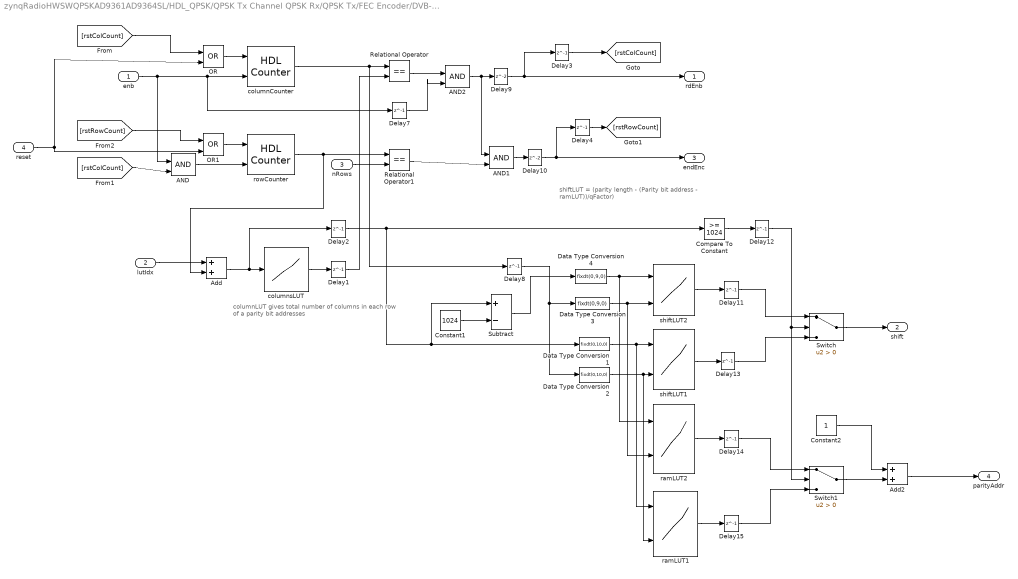
== system zynqRadioHWSWQPSKAD9361AD9364SL/HDL_QPSK/QPSK Tx Channel QPSK Rx/QPSK Tx/FEC Encoder/DVB-S2 LDPC Encoder/Parity Address Generator ==
  note: shiftLUT = (parity length - (Parity bit address -
      | ramLUT))/qFactor)
  note: columnLUT gives total number of columns
      | in each row of a parity bit addresses
  enb : Inport
  lutIdx : Inport  Port=2
  nRows : Inport  Port=3
  reset : Inport  Port=4
  AND : Logic  IconShape=distinctive  AllPortsSameDT=off  OutDataTypeStr=boolean
  AND1 : Logic  IconShape=distinctive  AllPortsSameDT=off  OutDataTypeStr=boolean
  AND2 : Logic  IconShape=distinctive  AllPortsSameDT=off  OutDataTypeStr=boolean
  Add : Sum  OutDataTypeStr=fixdt(0,11,0)
  Add2 : Sum  OutDataTypeStr=uint8
  Compare To Constant : simulink/Logic and Bit Operations/Compare To Constant  relop=>=  const=1024  OutDataTypeStr=boolean
  Constant1 : Constant  Value=1024  OutDataTypeStr=fixdt(0,11,0)  SampleTime=-1
  Constant2 : Constant  OutDataTypeStr=uint8  SampleTime=-1
  Data Type Conversion1 : DataTypeConversion  OutDataTypeStr=fixdt(0,10,0)  SaturateOnIntegerOverflow=off  RndMeth=Floor
  Data Type Conversion2 : DataTypeConversion  OutDataTypeStr=fixdt(0,10,0)  SaturateOnIntegerOverflow=off  RndMeth=Floor
  Data Type Conversion3 : DataTypeConversion  OutDataTypeStr=fixdt(0,9,0)  SaturateOnIntegerOverflow=off  RndMeth=Floor
  Data Type Conversion4 : DataTypeConversion  OutDataTypeStr=fixdt(0,9,0)  SaturateOnIntegerOverflow=off  RndMeth=Floor
  Delay1 : Delay  DelayLength=1  InitialCondition=0
  Delay10 : Delay
  Delay{2..4,7..8,11..15} (10 alike) : Delay  DelayLength=1
  Delay9 : Delay
  OR : Logic  Operator=OR  IconShape=distinctive  AllPortsSameDT=off  OutDataTypeStr=boolean
  OR1 : Logic  Operator=OR  IconShape=distinctive  AllPortsSameDT=off  OutDataTypeStr=boolean
  Relational Operator : RelationalOperator  Operator===  OutDataTypeStr=boolean  RndMeth=Simplest  InputSameDT=off
  Relational Operator1 : RelationalOperator  Operator===  OutDataTypeStr=boolean  RndMeth=Simplest  InputSameDT=off
  Subtract : Sum  Inputs=+-  OutDataTypeStr=fixdt(0,9,0)
  Switch : Switch  Criteria=u2 > Threshold  SaturateOnIntegerOverflow=off  InputSameDT=off
  Switch1 : Switch  Criteria=u2 > Threshold  SaturateOnIntegerOverflow=off  InputSameDT=off
  columnCounter : hdlsllib/Sources/HDL Counter  CountType=Count limited  CountInit=1  CountStep=1  CountMax=31  CountFromType=Initial value  CountFrom=1  CountResetPort=on  CountLoadPort=off  CountEnbPort=on  CountDirPort=off  CountHitOutputPort=off  CountDataType=Unsigned  CountWordLen=5  CountFracLen=0  CountSampTime=1
  columnsLUT : Lookup_n-D  NumberOfTableDimensions=1  BreakpointsSpecification=Even spacing  BreakpointsForDimension1=[1:20]  BreakpointsForDimension1FirstPoint=0  Table=columnSum  InterpMethod=Flat  RemoveProtectionInput=on  InternalRulePriority=Speed  OutDataTypeStr=fixdt(0,5,0)  RndMeth=Simplest
  ramLUT1 : Lookup_n-D  BreakpointsSpecification=Even spacing  BreakpointsForDimension1=[1:20]  BreakpointsForDimension2=[1:8]  BreakpointsForDimension1FirstPoint=0  BreakpointsForDimension1DataTypeStr=fixdt(0,10,0)  BreakpointsForDimension2DataTypeStr=fixdt(0,8,0)  Table=fi(ramLUT1,0,8,0)  TableDataTypeStr=Inherit: Inherit from 'Table data'  InterpMethod=Flat  DiagnosticForOutOfRangeInput=Warning  InternalRulePriority=Speed  OutDataTypeStr=Inherit: Inherit from 'Table data'  RndMeth=Simplest
      settings: InputPortMap=u0,u1
  ramLUT2 : Lookup_n-D  BreakpointsSpecification=Even spacing  BreakpointsForDimension1=[1:20]  BreakpointsForDimension2=[1:8]  BreakpointsForDimension1FirstPoint=0  BreakpointsForDimension1DataTypeStr=fixdt(0,9,0)  BreakpointsForDimension2DataTypeStr=fixdt(0,8,0)  Table=fi(ramLUT2,0,8,0)  TableDataTypeStr=Inherit: Inherit from 'Table data'  InterpMethod=Flat  DiagnosticForOutOfRangeInput=Warning  InternalRulePriority=Speed  OutDataTypeStr=Inherit: Inherit from 'Table data'  RndMeth=Simplest
      settings: InputPortMap=u0,u1
  rowCounter : hdlsllib/Sources/HDL Counter  CountType=Count limited  CountInit=1  CountStep=1  CountMax=162  CountFromType=Initial value  CountFrom=1  CountResetPort=on  CountLoadPort=off  CountEnbPort=on  CountDirPort=off  CountHitOutputPort=off  CountDataType=Unsigned  CountWordLen=8  CountFracLen=0  CountSampTime=1
  shiftLUT1 : Lookup_n-D  BreakpointsSpecification=Even spacing  BreakpointsForDimension1=[1:20]  BreakpointsForDimension2=[1:8]  BreakpointsForDimension1FirstPoint=0  BreakpointsForDimension1DataTypeStr=fixdt(0,10,0)  BreakpointsForDimension2DataTypeStr=fixdt(0,8,0)  Table=fi(shiftLUT1,0,9,0)  TableDataTypeStr=Inherit: Inherit from 'Table data'  InterpMethod=Flat  DiagnosticForOutOfRangeInput=Warning  InternalRulePriority=Speed  OutDataTypeStr=Inherit: Inherit from 'Table data'  RndMeth=Simplest
      settings: InputPortMap=u0,u1
  shiftLUT2 : Lookup_n-D  BreakpointsSpecification=Even spacing  BreakpointsForDimension1=[1:20]  BreakpointsForDimension2=[1:8]  BreakpointsForDimension1FirstPoint=0  BreakpointsForDimension1DataTypeStr=fixdt(0,9,0)  BreakpointsForDimension2DataTypeStr=fixdt(0,8,0)  Table=fi(shiftLUT2,0,9,0)  TableDataTypeStr=Inherit: Inherit from 'Table data'  InterpMethod=Flat  DiagnosticForOutOfRangeInput=Warning  InternalRulePriority=Speed  OutDataTypeStr=Inherit: Inherit from 'Table data'  RndMeth=Simplest
      settings: InputPortMap=u0,u1
  rdEnb : Outport
  shift : Outport  Port=2
  endEnc : Outport  Port=3
  parityAddr : Outport  Port=4
  wires:
  Add2/1 -> parityAddr/1
  Data Type Conversion2/1 -> shiftLUT1/2, ramLUT1/2
  Delay11/1 -> Switch/1
  nRows/1 -> Relational Operator1/2
  shiftLUT1/1 -> Delay13/1
  Delay14/1 -> Switch1/1
  ramLUT1/1 -> Delay15/1
  OR/1 -> columnCounter/1
  OR1/1 -> rowCounter/1
  Switch/1 -> shift/1
  Delay2/1 -> Compare To Constant/1, Data Type Conversion1/1, Subtract/1
  Delay15/1 -> Switch1/3
  Relational Operator/1 -> AND2/1
  Delay7/1 -> AND2/2
  Delay9/1 -> Delay3/1, rdEnb/1
  Delay4/1 -> [rstRowCount]
  columnCounter/1 -> Relational Operator/1, Delay8/1
  enb/1 -> Delay7/1, columnCounter/2, AND/1
  AND/1 -> rowCounter/2
  AND2/1 -> Delay9/1, AND1/1
  Data Type Conversion1/1 -> shiftLUT1/1, ramLUT1/1
  Compare To Constant/1 -> Delay12/1
  Delay12/1 -> Switch/2, Switch1/2
  lutIdx/1 -> Add/1
  [rstColCount] -> OR/1
  Delay3/1 -> [rstColCount]
  reset/1 -> OR/2, OR1/2
  AND1/1 -> Delay10/1
  Delay10/1 -> Delay4/1, endEnc/1
  Add/1 -> columnsLUT/1, Delay2/1
  Relational Operator1/1 -> AND1/2
  [rstColCount] -> AND/2
  Delay1/1 -> Relational Operator/2
  [rstRowCount] -> OR1/1
  columnsLUT/1 -> Delay1/1
  shiftLUT2/1 -> Delay11/1
  Constant2/1 -> Add2/1
  rowCounter/1 -> Add/2, Relational Operator1/1
  ramLUT2/1 -> Delay14/1
  Data Type Conversion4/1 -> ramLUT2/1, shiftLUT2/1
  Data Type Conversion3/1 -> ramLUT2/2, shiftLUT2/2
  Subtract/1 -> Data Type Conversion4/1
  Delay8/1 -> Data Type Conversion3/1, Data Type Conversion2/1
  Delay13/1 -> Switch/3
  Constant1/1 -> Subtract/2
  Switch1/1 -> Add2/2
